simulink model "X3_DecentralizedPD"  (R2024b)
settings: Solver=VariableStepAuto  StartTime=0.0  StopTime=20  RelTol=1e-3
libraries: dspinverses x1, Mako_Dynamics x1, g_block x1
settings Model: Creator=pinto  LastModifiedBy=pinto

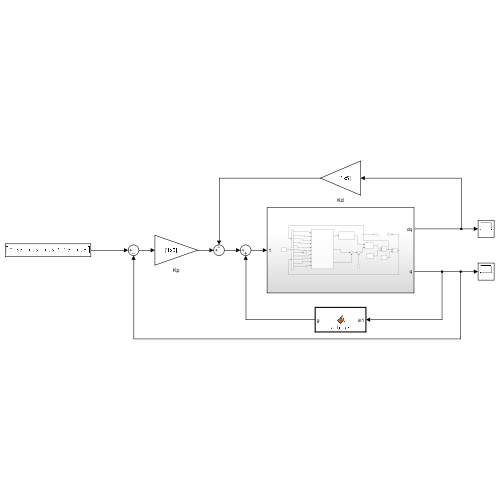
[thumbnail: Simulink's stored preview of the top-level diagram]
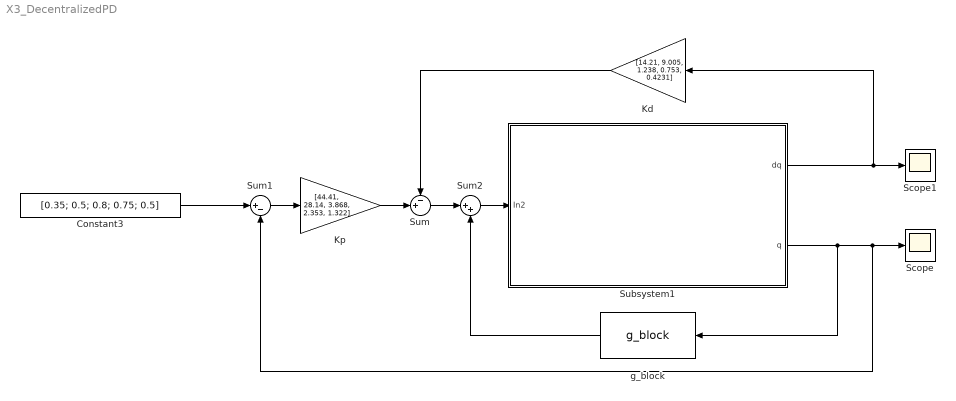
== system X3_DecentralizedPD ==
  Constant3 : Constant  Value=[0.35; 0.5; 0.8; 0.75; 0.5]
  Kd : Gain  Gain=[14.21, 9.005, 1.238, 0.753, 0.4231]
  Kp : Gain  Gain=[44.41, 28.14, 3.868, 2.353, 1.322]
  Scope : Scope
  Scope1 : Scope
  Subsystem1 : Subsystem
  Sum : Sum  Inputs=-+|
  Sum1 : Sum  Inputs=|+-
  Sum2 : Sum  Inputs=|++
  g_block : g_block/g_block  SystemSampleTime=-1  VariantActivationTime=update diagram  AllowFlexibleInterface=on  Latency=0  AutoFrameSizeCalculation=off
  wires:
  Kd/1 -> Sum/1
  Subsystem1/2(q) -> g_block/1, Sum1/2, Scope/1
  Kp/1 -> Sum/2
  Sum1/1 -> Kp/1
  Subsystem1/1(dq) -> Kd/1, Scope1/1
  Constant3/1 -> Sum1/1
  Sum/1 -> Sum2/1
  Sum2/1 -> Subsystem1/1(In2)
  g_block/1 -> Sum2/2

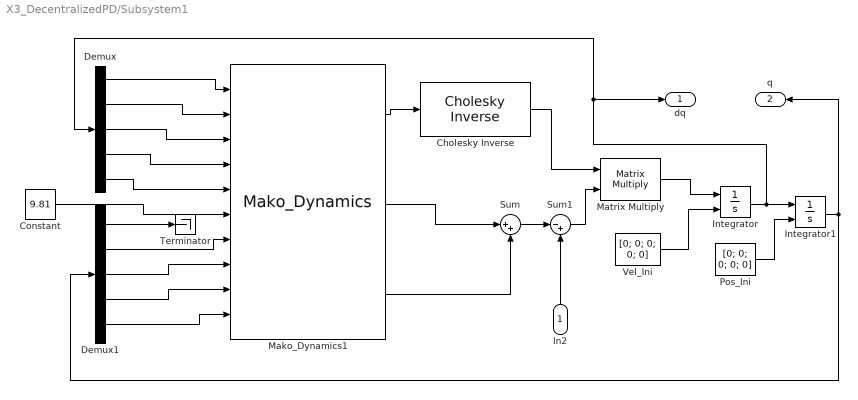
== system X3_DecentralizedPD/Subsystem1 ==
  In2 : Inport
  Cholesky Inverse : dspinverses/Cholesky Inverse  errmode=Warning
  Constant : Constant  Value=9.81
  Demux : Demux  Outputs=5
  Demux1 : Demux  Outputs=5
  Integrator : Integrator  InitialConditionSource=external  InitialCondition=[0.01, 0.01, 0.01]
  Integrator1 : Integrator  InitialConditionSource=external  InitialCondition=[0.01, 0.01, 0.01]
  Mako_Dynamics1 : Mako_Dynamics/Mako_Dynamics  SystemSampleTime=-1  VariantActivationTime=update diagram  AllowFlexibleInterface=on  Latency=0  AutoFrameSizeCalculation=off
  Matrix Multiply : Product  Multiplication=Matrix(*)
  Pos_Ini : Constant  Value=[0; 0; 0; 0; 0]
  Sum : Sum  Inputs=|++
  Sum1 : Sum  Inputs=|-+
  Terminator : Terminator
  Vel_Ini : Constant  Value=[0; 0; 0; 0; 0]
  dq : Outport
  q : Outport  Port=2
  wires:
  Sum/1 -> Sum1/1
  Mako_Dynamics1/3 -> Sum/2
  Demux/3 -> Mako_Dynamics1/3
  Integrator/1 -> Integrator1/1, Demux/1, dq/1
  Matrix Multiply/1 -> Integrator/1
  Demux/4 -> Mako_Dynamics1/4
  Demux/2 -> Mako_Dynamics1/2
  Pos_Ini/1 -> Integrator1/2
  Integrator1/1 -> q/1, Demux1/1
  Mako_Dynamics1/1 -> Cholesky Inverse/1
  Cholesky Inverse/1 -> Matrix Multiply/1
  Vel_Ini/1 -> Integrator/2
  Sum1/1 -> Matrix Multiply/2
  Demux/1 -> Mako_Dynamics1/1
  In2/1 -> Sum1/2
  Mako_Dynamics1/2 -> Sum/1
  Demux/5 -> Mako_Dynamics1/5
  Demux1/1 -> Terminator/1
  Constant/1 -> Mako_Dynamics1/6
  Demux1/2 -> Mako_Dynamics1/7
  Demux1/3 -> Mako_Dynamics1/8
  Demux1/4 -> Mako_Dynamics1/9
  Demux1/5 -> Mako_Dynamics1/10
